simulink model "One_level_boost_igbt"  (R2022a)
settings: Solver=VariableStepAuto  StartTime=0.0  StopTime=10  MaxStep=10e-6  RelTol=1e-3
libraries: spsSeriesRLCBranchLib x3, spsCurrentMeasurementLib x1, spsDiodeLib x1, spsIGBTLib x1, spsDCVoltageSourceLib x1, spsVoltageMeasurementLib x1, spspowerguiLib x1
settings Model: Creator=Andris  LastModifiedBy=Andris

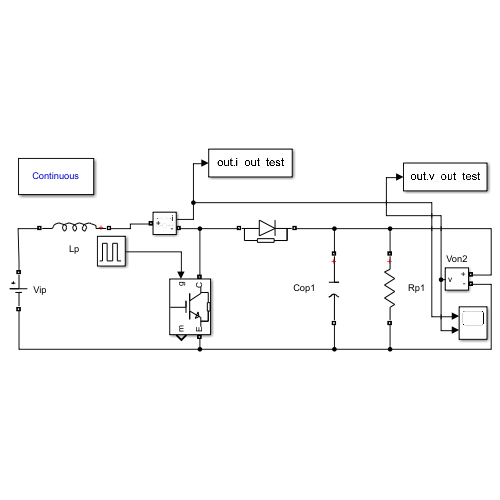
[thumbnail: Simulink's stored preview of the top-level diagram]
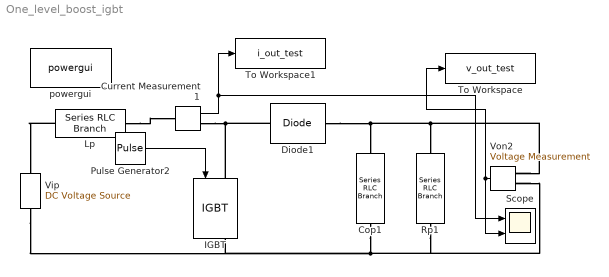
== system One_level_boost_igbt ==
  Cop1 : spsSeriesRLCBranchLib/Series RLC Branch  LConnTagsString=__new0  RConnTagsString=__new0  BranchType=C  Resistance=1  Inductance=1e-3  SetiL0=off  InitialCurrent=0  Capacitance=0.001  Setx0=off  InitialVoltage=Vop1  Measurements=None
  Current Measurement1 : spsCurrentMeasurementLib/Current Measurement  PhasorSimulation=off  OutputType=Complex  PSBequivalent=0
  Diode1 : spsDiodeLib/Diode  Ron=0.033  Lon=0  Vf=0.8  IC=0  UseSnubber=off  Rs=100000  Cs=inf  Measurements=off
  IGBT : spsIGBTLib/IGBT  Ron=0.25  Lon=0  Vf=0.8  Tf=1e-6  Tt=2e-6  IC=0  Rs=1e5  Cs=inf  Measurements=on
  Lp : spsSeriesRLCBranchLib/Series RLC Branch  LConnTagsString=__new0  RConnTagsString=__new0  BranchType=L  Resistance=1  Inductance=0.001  SetiL0=off  InitialCurrent=0  Capacitance=1e-6  Setx0=off  InitialVoltage=0  Measurements=None
  Pulse Generator2 : DiscretePulseGenerator  PulseType=Time based  Period=1/48229  PulseWidth=50  PhaseDelay=(1/48229)*(29/100)
  Rp1 : spsSeriesRLCBranchLib/Series RLC Branch  LConnTagsString=__new0  RConnTagsString=__new0  BranchType=R  Resistance=100  Inductance=1e-3  SetiL0=off  InitialCurrent=0  Capacitance=1e-6  Setx0=off  InitialVoltage=0  Measurements=None
  Scope : Scope  NumInputPorts=2
  To Workspace : ToWorkspace  VariableName=v_out_test  SampleTime=0.001
      settings: MaxDataPoints=8000  Save2DSignal=2-D array (concatenate along first dimension)
  To Workspace1 : ToWorkspace  VariableName=i_out_test  SampleTime=0.001
      settings: MaxDataPoints=8000  Save2DSignal=2-D array (concatenate along first dimension)
  Vip : spsDCVoltageSourceLib/DC Voltage Source  Amplitude=5  Measurements=None
  Von2 : spsVoltageMeasurementLib/Voltage Measurement  PhasorSimulation=off  OutputType=Complex  PSBequivalent=0
  powergui : spspowerguiLib/powergui  Priority=1  SimulationMode=Continuous  SampleTime=50e-6  frequency=60  Iterations=50  frequencyindice=0  Pbase=100e6  ErrMax=1e-4  UnitsV=kV  UnitsW=MW  buscounter=0  FunctionMessages=off  echomessages=off  EnableUseOfTLC=off  CurrentSourceSwitches=off  DisableSnubberDevices=off  DisableRonSwitches=off  DisableVfSwitches=off  DisplayEquations=off  AutomaticDiscreteSolvers=off  SolverType=Tustin/Backward Euler (TBE)  Interpol=off  ExternalGateDelay=off  methode=off  Ts=100  x0status=blocks  SPID=on  SwTol=0  HookPort=off  NonlinearTolerance=1e-4  nMaxIteration=100  ContinueOnMaxIteration=off  RestoreLinks=warning  ResistiveCurrentMeasurement=off  Frange=[0:2:500]  Ylog=off  Xlog=on  ShowGrid=off  save=off  variable=ZData  structure=0  ZoomFFT=off  StartTime=0.0  cycles=1  DisplayStyle=1  fundamental=60  FreqAxis=off  MaxFrequency=1000  frequencyindicesteady=1  RmsSteady=1  display=off
  wires:
  Von2/1 -> To Workspace/1, Scope/2
  Current Measurement1/1 -> Scope/1, To Workspace1/1
  Pulse Generator2/1 -> IGBT/1
  connections:
  Von2/LConn2 -- Rp1/RConn1 -- Cop1/RConn1 -- IGBT/RConn1 -- Vip/LConn1
  Lp/RConn1 -- Vip/RConn1
  Current Measurement1/RConn1 -- IGBT/LConn1 -- Diode1/LConn1
  Lp/LConn1 -- Current Measurement1/LConn1
  Von2/LConn1 -- Diode1/RConn1 -- Cop1/LConn1 -- Rp1/LConn1
